simulink model "Project"  (R2018a)
settings: Solver=VariableStepAuto  StartTime=0  StopTime=1  FixedStep=Ts  RelTol=1e-3  AbsTol=1e-3
PreLoadFcn:
  | Ts=2e-6;
  | Ts_Control=100e-6;
undefined symbols (not defined in the file): Hydride, Metal, Nickel, Vnom_dc
libraries: powerlib x111, powerlib_extras x45, simulink x32, powerlib_meascontrol x13, dspswit3 x9, electricdrivelib x2, re_lib x2
(part 1 of 4)
Description:
  | Copyright 2008-2011 The MathWorks, Inc.
settings Model: FPTRunName=Active  ExtModeTrigMode=oneshot  ExtModeArmWhenConnect=off  ExtModeAutoUpdateStatusClock=off  Creator=MathWorks  LastModifiedBy=Lenovo
settings SolverCC: AutoScaleAbsTol=off
settings DataIOCC: SaveFormat=Array  SignalLoggingSaveFormat=ModelDataLogs  SaveOutput=off  SaveTime=off  SignalLoggingName=sigsOut
settings OptimizationCC: BlockReduction=off  BooleanDataType=off  ExpressionDepthLimit=2147483647  InitFltsAndDblsToZero=on  EfficientMapNaN2IntZero=off  LifeSpan=inf
settings DebuggingCC: SaveWithParameterizedLinksMsg=none  UnderspecifiedInitializationDetection=Classic  MergeDetectMultiDrivingBlocksExec=none  CheckExecutionContextPreStartOutputMsg=on  CheckExecutionContextRuntimeOutputMsg=on  SignalResolutionControl=TryResolveAllWithWarning  MultiTaskDSMMsg=warning  MultiTaskCondExecSysMsg=none  FcnCallInpInsideContextMsg=warning  StateNameClashWarn=warning  SFUnexpectedBacktrackingDiag=warning  SFNoUnconditionalDefaultTransitionDiag=warning  SFExecutionAtInitializationDiag=none
settings HardwareCC: ProdBitPerPointer=32  ProdBitPerSizeT=32  ProdBitPerPtrDiffT=32  ProdLargestAtomicFloat=None  ProdIntDivRoundTo=Undefined  ProdEndianess=Unspecified  ProdWordSize=32  ProdHWDeviceType=32-bit Generic  TargetUnknown=on
settings ModelReferenceCC: PropagateSignalLabelsOutOfModel=off
settings CodeAppCC: StateflowObjectComments=on
settings GRTTargetCC: TargetFcnLib=ansi_tfl_tmw.mat  TargetLangStandard=C89/C90 (ANSI)  GeneratePreprocessorConditionals=Disable all  CombineOutputUpdateFcns=off  GRTInterface=on
settings ConfigComp: CovMetricSettings=dw  CovHtmlReporting=on  CovSaveCumulativeToWorkspaceVar=on  CovSaveSingleToWorkspaceVar=on  CovExternalEMLEnable=off
settings SimscapeCC: SimscapeNormalizeSystem=off

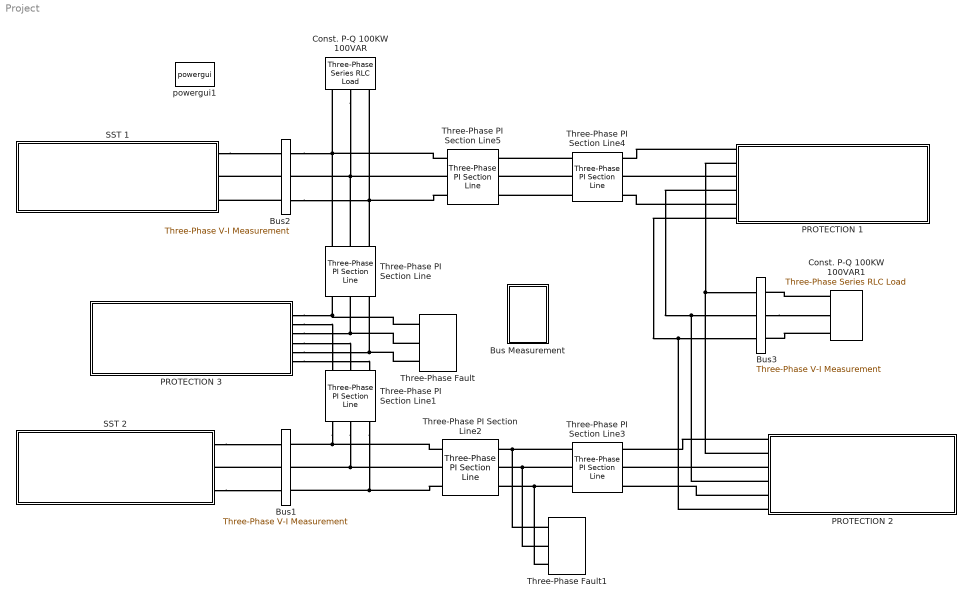
== system Project ==
  Bus Measurement : Subsystem
  Bus1 : powerlib/Measurements/Three-Phase V-I Measurement  VoltageMeasurement=phase-to-phase  SetLabelV=on  LabelV=Bus1_V  Vpu=off  VpuLL=off  CurrentMeasurement=yes  SetLabelI=on  LabelI=Bus1_I  Ipu=off  Pbase=100e6  Vbase=500e3  OutputType=Complex  PhasorSimulation=off  PSBequivalent=0
  Bus2 : powerlib/Measurements/Three-Phase V-I Measurement  VoltageMeasurement=phase-to-phase  SetLabelV=on  LabelV=Bus2_V  Vpu=off  VpuLL=off  CurrentMeasurement=yes  SetLabelI=on  LabelI=Bus2_I  Ipu=off  Pbase=100e6  Vbase=500e3  OutputType=Complex  PhasorSimulation=off  PSBequivalent=0
  Bus3 : powerlib/Measurements/Three-Phase V-I Measurement  VoltageMeasurement=phase-to-phase  SetLabelV=on  LabelV=Bus3_V  Vpu=off  VpuLL=off  CurrentMeasurement=yes  SetLabelI=on  LabelI=Bus3_I  Ipu=off  Pbase=100e6  Vbase=500e3  OutputType=Complex  PhasorSimulation=off  PSBequivalent=0
  Const. P-Q 100KW 100VAR : powerlib/Elements/Three-Phase Series RLC Load  LConnTagsString=A|B|C  Configuration=Y (grounded)  NominalVoltage=380  Vabc=[1e3 1e3 1e3]  Vabcp=[1e3 1e3 1e3]  NominalFrequency=60  UnbalancedPower=off  ActivePower=100e3  InductivePower=100  CapacitivePower=100  Pabc=[10e3 9e3 11e3]  QLabc=[100 90 110]  QCabc=[100 90 110]  Pabcp=[10e3 9e3 11e3]  QLabcp=[100 90 110]  QCabcp=[100 90 110]  Measurements=None  LoadType=constant PQ
  Const. P-Q 100KW 100VAR1 : powerlib/Elements/Three-Phase Series RLC Load  LConnTagsString=A|B|C  Configuration=Y (grounded)  NominalVoltage=380  Vabc=[1e3 1e3 1e3]  Vabcp=[1e3 1e3 1e3]  NominalFrequency=60  UnbalancedPower=off  ActivePower=100e3  InductivePower=100  CapacitivePower=100  Pabc=[10e3 9e3 11e3]  QLabc=[100 90 110]  QCabc=[100 90 110]  Pabcp=[10e3 9e3 11e3]  QLabcp=[100 90 110]  QCabcp=[100 90 110]  Measurements=None  LoadType=constant PQ
  PROTECTION 1 : Subsystem
  PROTECTION 2 : Subsystem
  PROTECTION 3 : Subsystem
  SST 1 : Subsystem
  SST 2 : Subsystem
  Three-Phase PI Section Line{,1..5} (6 alike) : powerlib/Elements/Three-Phase PI Section Line  LConnTagsString=a|b|c  RConnTagsString=A|B|C  Frequency=60  Resistances=[ 0.01273 0.3864]  Inductances="[ 0.9337e-3  4.1264e-3]"  Capacitances=[12.74e-9 7.751e-9]  Length=1
      settings: SourceProductName=Simscape Power Systems
  Three-Phase Fault : powerlib/Elements/Three-Phase Fault  InitialStates=0  FaultA=on  FaultB=on  FaultC=on  GroundFault=on  SwitchTimes=[0.5]  External=off  SwitchStatus=NaN  FaultResistance=0.001  GroundResistance=0.01  SnubberResistance=1e6  SnubberCapacitance=inf  Measurements=None
  Three-Phase Fault1 : powerlib/Elements/Three-Phase Fault  InitialStates=0  FaultA=on  FaultB=on  FaultC=on  GroundFault=on  SwitchTimes=[0.8 0.9]  External=off  SwitchStatus=NaN  FaultResistance=0.001  GroundResistance=0.01  SnubberResistance=1e6  SnubberCapacitance=inf  Measurements=None
  powergui1 : powerlib/powergui  Priority=2  SimulationMode=Discrete  SampleTime=5e-6  frequency=60  Iterations=50  frequencyindice=0  Pbase=100e6  ErrMax=1e-4  UnitsV=kV  UnitsW=MW  buscounter=0  FunctionMessages=off  echomessages=on  EnableUseOfTLC=off  CurrentSourceSwitches=off  DisableSnubberDevices=off  DisableRonSwitches=off  DisableVfSwitches=off  DisplayEquations=off  SolverType=Tustin/Backward Euler (TBE)  Interpol=off  ExternalGateDelay=off  methode=off  Ts=100  x0status=blocks  SPID=off  SwTol=0  HookPort=off  RestoreLinks=warning  ResistiveCurrentMeasurement=off  Frange=[0:2:500]  Ylog=off  Xlog=on  ShowGrid=off  save=off  variable=ZData  structure=psbbridges_str  ZoomFFT=on  StartTime=0.1-2/50  cycles=2  DisplayStyle=off  fundamental=50  FreqAxis=off  MaxFrequency=7000  frequencyindicesteady=1  RmsSteady=1  display=off
  connections:
  Bus2/RConn1 -- Three-Phase PI Section Line/LConn1 -- Three-Phase PI Section Line5/RConn1 -- Const. P-Q 100KW 100VAR/LConn1
  Const. P-Q 100KW 100VAR/LConn2 -- Three-Phase PI Section Line/LConn2 -- Three-Phase PI Section Line5/RConn2 -- Bus2/RConn2
  Bus2/RConn3 -- Three-Phase PI Section Line/LConn3 -- Three-Phase PI Section Line5/RConn3 -- Const. P-Q 100KW 100VAR/LConn3
  SST 1/LConn1 -- Bus2/LConn1
  Bus2/LConn2 -- SST 1/LConn2
  Bus2/LConn3 -- SST 1/LConn3
  SST 2/LConn1 -- Bus1/LConn1
  Bus1/LConn2 -- SST 2/LConn2
  SST 2/LConn3 -- Bus1/LConn3
  Three-Phase PI Section Line1/RConn1 -- Three-Phase PI Section Line2/RConn1 -- Bus1/RConn1
  Three-Phase PI Section Line1/RConn2 -- Three-Phase PI Section Line2/RConn2 -- Bus1/RConn2
  Three-Phase PI Section Line1/RConn3 -- Three-Phase PI Section Line2/RConn3 -- Bus1/RConn3
  Const. P-Q 100KW 100VAR1/LConn1 -- Bus3/RConn1
  Bus3/RConn2 -- Const. P-Q 100KW 100VAR1/LConn2
  Const. P-Q 100KW 100VAR1/LConn3 -- Bus3/RConn3
  Three-Phase PI Section Line4/RConn1 -- Three-Phase PI Section Line5/LConn1
  Three-Phase PI Section Line4/RConn2 -- Three-Phase PI Section Line5/LConn2
  Three-Phase PI Section Line4/RConn3 -- Three-Phase PI Section Line5/LConn3
  Three-Phase PI Section Line3/RConn1 -- Three-Phase Fault1/LConn1 -- Three-Phase PI Section Line2/LConn1
  Three-Phase PI Section Line3/RConn2 -- Three-Phase Fault1/LConn2 -- Three-Phase PI Section Line2/LConn2
  Three-Phase PI Section Line3/RConn3 -- Three-Phase PI Section Line2/LConn3 -- Three-Phase Fault1/LConn3
  PROTECTION 1/LConn1 -- Three-Phase PI Section Line4/LConn1
  PROTECTION 1/LConn3 -- Three-Phase PI Section Line4/LConn2
  PROTECTION 1/LConn5 -- Three-Phase PI Section Line4/LConn3
  PROTECTION 1/LConn2 -- PROTECTION 2/LConn2 -- Bus3/LConn1
  PROTECTION 1/LConn4 -- PROTECTION 2/LConn4 -- Bus3/LConn2
  PROTECTION 1/LConn6 -- PROTECTION 2/LConn6 -- Bus3/LConn3
  PROTECTION 3/LConn1 -- Three-Phase Fault/LConn1 -- Three-Phase PI Section Line/RConn1
  PROTECTION 3/LConn3 -- Three-Phase Fault/LConn2 -- Three-Phase PI Section Line/RConn2
  PROTECTION 3/LConn5 -- Three-Phase Fault/LConn3 -- Three-Phase PI Section Line/RConn3
  PROTECTION 3/LConn2 -- Three-Phase PI Section Line1/LConn1
  PROTECTION 3/LConn4 -- Three-Phase PI Section Line1/LConn2
  PROTECTION 3/LConn6 -- Three-Phase PI Section Line1/LConn3
  PROTECTION 2/LConn1 -- Three-Phase PI Section Line3/LConn1
  PROTECTION 2/LConn3 -- Three-Phase PI Section Line3/LConn2
  PROTECTION 2/LConn5 -- Three-Phase PI Section Line3/LConn3

== system Project/Bus Measurement ==
  Scope{,1..5} (6 alike) : Scope
  wires:
  [Bus3_V] -> Scope4/1
  [Bus2_I] -> Scope3/1
  [Bus2_V] -> Scope2/1
  [Bus1_I] -> Scope1/1
  [Bus3_I] -> Scope5/1
  [Bus1_V] -> Scope/1

== system Project/PROTECTION 1 ==
  Current Measurement : powerlib/Measurements/Current Measurement  PhasorSimulation=off  OutputType=Complex  PSBequivalent=0
  Current Measurement1 : powerlib/Measurements/Current Measurement  PhasorSimulation=off  OutputType=Complex  PSBequivalent=0
  Current Measurement2 : powerlib/Measurements/Current Measurement  PhasorSimulation=off  OutputType=Complex  PSBequivalent=0
  overcurrent Fid : Subsystem
  overcurrent Fid1 : Subsystem
  overcurrent Fid2 : Subsystem
  overcurrent relay1 : Subsystem
  overcurrent relay2 : Subsystem
  overcurrent relay3 : Subsystem
  Conn1 : PMIOPort  Side=Left
  Conn2 : PMIOPort  Port=2  Side=Left
  Conn3 : PMIOPort  Port=3  Side=Left
  Conn4 : PMIOPort  Port=4  Side=Left
  Conn5 : PMIOPort  Port=5  Side=Left
  Conn6 : PMIOPort  Port=6  Side=Left
  wires:
  overcurrent relay1/1("CB control signal ") -> overcurrent Fid/1(In_Rly)
  overcurrent relay2/1("CB control signal ") -> overcurrent Fid2/1(In_Rly)
  overcurrent relay3/1("CB control signal ") -> overcurrent Fid1/1(In_Rly)
  Current Measurement/1 -> overcurrent relay1/1(Current)
  Current Measurement1/1 -> overcurrent relay2/1(Current)
  Current Measurement2/1 -> overcurrent relay3/1(Current)
  connections:
  Current Measurement2/LConn1 -- Conn5/RConn1
  overcurrent Fid1/LConn2 -- Conn6/RConn1
  overcurrent Fid/LConn2 -- Conn2/RConn1
  Current Measurement1/LConn1 -- Conn3/RConn1
  Current Measurement/LConn1 -- Conn1/RConn1
  Current Measurement/RConn1 -- overcurrent Fid/LConn1
  Current Measurement1/RConn1 -- overcurrent Fid2/LConn1
  Conn4/RConn1 -- overcurrent Fid2/LConn2
  Current Measurement2/RConn1 -- overcurrent Fid1/LConn1

== system Project/PROTECTION 2 ==
  Current Measurement : powerlib/Measurements/Current Measurement  PhasorSimulation=off  OutputType=Complex  PSBequivalent=0
  Current Measurement1 : powerlib/Measurements/Current Measurement  PhasorSimulation=off  OutputType=Complex  PSBequivalent=0
  Current Measurement2 : powerlib/Measurements/Current Measurement  PhasorSimulation=off  OutputType=Complex  PSBequivalent=0
  overcurrent Fid : Subsystem
  overcurrent Fid1 : Subsystem
  overcurrent Fid2 : Subsystem
  overcurrent relay1 : Subsystem
  overcurrent relay2 : Subsystem
  overcurrent relay3 : Subsystem
  Conn1 : PMIOPort  Side=Left
  Conn2 : PMIOPort  Port=2  Side=Left
  Conn3 : PMIOPort  Port=3  Side=Left
  Conn4 : PMIOPort  Port=4  Side=Left
  Conn5 : PMIOPort  Port=5  Side=Left
  Conn6 : PMIOPort  Port=6  Side=Left
  wires:
  Current Measurement1/1 -> overcurrent relay2/1(Current)
  overcurrent relay2/1("CB control signal ") -> overcurrent Fid2/1(In_Rly)
  Current Measurement2/1 -> overcurrent relay3/1(Current)
  overcurrent relay3/1("CB control signal ") -> overcurrent Fid1/1(In_Rly)
  Current Measurement/1 -> overcurrent relay1/1(Current)
  overcurrent relay1/1("CB control signal ") -> overcurrent Fid/1(In_Rly)
  connections:
  Current Measurement2/RConn1 -- overcurrent Fid1/LConn1
  overcurrent Fid1/LConn2 -- Conn6/RConn1
  Current Measurement/RConn1 -- overcurrent Fid/LConn1
  Current Measurement2/LConn1 -- Conn5/RConn1
  Current Measurement1/LConn1 -- Conn3/RConn1
  Conn4/RConn1 -- overcurrent Fid2/LConn2
  Current Measurement/LConn1 -- Conn1/RConn1
  Current Measurement1/RConn1 -- overcurrent Fid2/LConn1
  overcurrent Fid/LConn2 -- Conn2/RConn1

== system Project/PROTECTION 3 ==
  Current Measurement : powerlib/Measurements/Current Measurement  PhasorSimulation=off  OutputType=Complex  PSBequivalent=0
  Current Measurement1 : powerlib/Measurements/Current Measurement  PhasorSimulation=off  OutputType=Complex  PSBequivalent=0
  Current Measurement2 : powerlib/Measurements/Current Measurement  PhasorSimulation=off  OutputType=Complex  PSBequivalent=0
  Scope : Scope
  overcurrent Fid : Subsystem
  overcurrent Fid1 : Subsystem
  overcurrent Fid2 : Subsystem
  overcurrent relay1 : Subsystem
  overcurrent relay2 : Subsystem
  overcurrent relay3 : Subsystem
  Conn1 : PMIOPort  Side=Left
  Conn2 : PMIOPort  Port=2  Side=Left
  Conn3 : PMIOPort  Port=3  Side=Left
  Conn4 : PMIOPort  Port=4  Side=Left
  Conn5 : PMIOPort  Port=5  Side=Left
  Conn6 : PMIOPort  Port=6  Side=Left
  wires:
  Current Measurement1/1 -> overcurrent relay2/1(Current)
  overcurrent relay2/1("CB control signal ") -> overcurrent Fid2/1(In_Rly)
  Current Measurement2/1 -> overcurrent relay3/1(Current)
  overcurrent relay3/1("CB control signal ") -> overcurrent Fid1/1(In_Rly)
  Current Measurement/1 -> Scope/1, overcurrent relay1/1(Current)
  overcurrent relay1/1("CB control signal ") -> overcurrent Fid/1(In_Rly)
  connections:
  Current Measurement2/RConn1 -- overcurrent Fid1/LConn1
  overcurrent Fid1/LConn2 -- Conn6/RConn1
  Current Measurement/RConn1 -- overcurrent Fid/LConn1
  Current Measurement2/LConn1 -- Conn5/RConn1
  Current Measurement1/LConn1 -- Conn3/RConn1
  Conn4/RConn1 -- overcurrent Fid2/LConn2
  Current Measurement/LConn1 -- Conn1/RConn1
  Current Measurement1/RConn1 -- overcurrent Fid2/LConn1
  overcurrent Fid/LConn2 -- Conn2/RConn1

== system Project/SST 1 ==
  note: 1=SST
  note: 0=PV
  "6.2 kV, 60 Hz " : powerlib/Electrical Sources/Three-Phase Source  InternalConnection=Yg  VoltagePhases=off  Voltage=6.2e3  PhaseAngle=0  Voltage_phases=[25e3 25e3 25e3]/sqrt(3)  PhaseAngles_phases=[0 -120 +120]  Frequency=60  NonIdealSource=on  SpecifyImpedance=off  Resistance=25e3^2/10e6/5  Inductance=0  ShortCircuitLevel=1e6  BaseVoltage=6.2e3  XRratio=5  BusType=swing  Pref=0  Qref=0  Prefabc=[10e3, 10e3, 10e3]  Qrefabc=[0, 0, 0]  Qmin=-inf  Qmax=inf
  AC-DC Conversion : Subsystem
  Battery (DESD) : Subsystem
  C1 : powerlib/Elements/Parallel RLC Branch  LConnTagsString=a  RConnTagsString=__new0  BranchType=C  Resistance=inf  Inductance=inf  SetiL0=off  InitialCurrent=0  Capacitance=1800e-06  Setx0=off  InitialVoltage=0  Measurements=None
  C2 : powerlib/Elements/Parallel RLC Branch  LConnTagsString=a  RConnTagsString=__new0  BranchType=C  Resistance=inf  Inductance=inf  SetiL0=off  InitialCurrent=0  Capacitance=80e-3  Setx0=off  InitialVoltage=0  Measurements=None
  Constant : Constant
  DC-AC Conversion : Subsystem
  DC-DC Isolation : Subsystem
  PV (DRER) : Subsystem
  Switch : Subsystem
  a : PMIOPort  Side=Left
  b : PMIOPort  Port=2  Side=Left
  c : PMIOPort  Port=3  Side=Left
  wires:
  Constant/1 -> Switch/1(In1)
  connections:
  AC-DC Conversion/RConn1 -- C1/LConn1 -- DC-DC Isolation/RConn1
  "6.2 kV, 60 Hz "/RConn2 -- AC-DC Conversion/LConn2
  c/RConn1 -- DC-AC Conversion/LConn3
  DC-AC Conversion/RConn2 -- PV (DRER)/LConn2 -- DC-DC Isolation/LConn2 -- Battery (DESD)/LConn1 -- C2/RConn1
  "6.2 kV, 60 Hz "/RConn3 -- AC-DC Conversion/LConn3
  Switch/LConn1 -- PV (DRER)/LConn1
  C2/LConn1 -- Switch/RConn1 -- Battery (DESD)/RConn1 -- DC-AC Conversion/RConn1
  "6.2 kV, 60 Hz "/RConn1 -- AC-DC Conversion/LConn1
  DC-DC Isolation/RConn2 -- C1/RConn1 -- AC-DC Conversion/RConn2
  Switch/LConn2 -- DC-DC Isolation/LConn1
  DC-AC Conversion/LConn1 -- a/RConn1
  b/RConn1 -- DC-AC Conversion/LConn2

== system Project/SST 2 ==
  note: 1=SST
  note: 0=PV
  "6.2 kV, 60 Hz 1" : powerlib/Electrical Sources/Three-Phase Source  InternalConnection=Yg  VoltagePhases=off  Voltage=6.2e3  PhaseAngle=0  Voltage_phases=[25e3 25e3 25e3]/sqrt(3)  PhaseAngles_phases=[0 -120 +120]  Frequency=60  NonIdealSource=on  SpecifyImpedance=off  Resistance=25e3^2/10e6/5  Inductance=0  ShortCircuitLevel=1e6  BaseVoltage=6.2e3  XRratio=5  BusType=swing  Pref=0  Qref=0  Prefabc=[10e3, 10e3, 10e3]  Qrefabc=[0, 0, 0]  Qmin=-inf  Qmax=inf
  AC-DC Conversion1 : Subsystem
  Battery (DESD)1 : Subsystem
  C3 : powerlib/Elements/Parallel RLC Branch  LConnTagsString=a  RConnTagsString=__new0  BranchType=C  Resistance=inf  Inductance=inf  SetiL0=off  InitialCurrent=0  Capacitance=1800e-06  Setx0=off  InitialVoltage=0  Measurements=None
  C4 : powerlib/Elements/Parallel RLC Branch  LConnTagsString=a  RConnTagsString=__new0  BranchType=C  Resistance=inf  Inductance=inf  SetiL0=off  InitialCurrent=0  Capacitance=80e-3  Setx0=off  InitialVoltage=0  Measurements=None
  Constant1 : Constant
  DC-AC Conversion1 : Subsystem
  DC-DC Isolation1 : Subsystem
  PV (DRER)1 : Subsystem
  Switch1 : Subsystem
  a : PMIOPort  Side=Left
  b : PMIOPort  Port=2  Side=Left
  c : PMIOPort  Port=3  Side=Left
  wires:
  Constant1/1 -> Switch1/1(In1)
  connections:
  C4/RConn1 -- DC-AC Conversion1/RConn2 -- PV (DRER)1/LConn2 -- DC-DC Isolation1/LConn2 -- Battery (DESD)1/LConn1
  AC-DC Conversion1/LConn3 -- "6.2 kV, 60 Hz 1"/RConn3
  "6.2 kV, 60 Hz 1"/RConn2 -- AC-DC Conversion1/LConn2
  Switch1/LConn2 -- DC-DC Isolation1/LConn1
  AC-DC Conversion1/RConn2 -- DC-DC Isolation1/RConn2 -- C3/RConn1
  Switch1/LConn1 -- PV (DRER)1/LConn1
  "6.2 kV, 60 Hz 1"/RConn1 -- AC-DC Conversion1/LConn1
  DC-AC Conversion1/RConn1 -- C4/LConn1 -- Switch1/RConn1 -- Battery (DESD)1/RConn1
  DC-DC Isolation1/RConn1 -- AC-DC Conversion1/RConn1 -- C3/LConn1
  DC-AC Conversion1/LConn1 -- a/RConn1
  DC-AC Conversion1/LConn3 -- c/RConn1
  b/RConn1 -- DC-AC Conversion1/LConn2

== system Project/PROTECTION 1/overcurrent Fid ==
  In_Rly : Inport
  Diode1 : powerlib/Power Electronics/Diode  Ron=0.001  Lon=0  Vf=1  IC=150  UseSnubber=0  Rs=500  Cs=250e-9  Measurements=off
  Diode2 : powerlib/Power Electronics/Diode  Ron=0.001  Lon=0  Vf=1  IC=150  UseSnubber=0  Rs=500  Cs=250e-9  Measurements=off
  IGBT1 : powerlib/Power Electronics/IGBT  Ron=0.001  Lon=100e-6  Vf=3  Tf=1e-6  Tt=2e-6  IC=150  Rs=1e5  Cs=inf  Measurements=on
  IGBT2 : powerlib/Power Electronics/IGBT  Ron=0.001  Lon=100e-6  Vf=3  Tf=1e-6  Tt=2e-6  IC=150  Rs=1e5  Cs=inf  Measurements=on
  Scope : Scope  NumInputPorts=2
  In : PMIOPort  Tag=PMCPort  Side=Left
  Out : PMIOPort  Tag=PMCPort  Port=2  Side=Left
  wires:
  IGBT1/1 -> [igbt1]
  [igbt1] -> Scope/2
  In_Rly/1 -> IGBT1/1, IGBT2/1
  IGBT2/1 -> [igbt]
  [igbt] -> Scope/1
  connections:
  IGBT2/RConn1 -- Diode2/LConn1 -- IGBT1/RConn1 -- Diode1/LConn1
  In/RConn1 -- Diode1/RConn1 -- IGBT2/LConn1
  Out/RConn1 -- Diode2/RConn1 -- IGBT1/LConn1

== system Project/PROTECTION 1/overcurrent Fid1 ==
  In_Rly : Inport
  Diode1 : powerlib/Power Electronics/Diode  Ron=0.001  Lon=0  Vf=1  IC=150  UseSnubber=0  Rs=500  Cs=250e-9  Measurements=off
  Diode2 : powerlib/Power Electronics/Diode  Ron=0.001  Lon=0  Vf=1  IC=150  UseSnubber=0  Rs=500  Cs=250e-9  Measurements=off
  IGBT1 : powerlib/Power Electronics/IGBT  Ron=0.001  Lon=100e-6  Vf=3  Tf=1e-6  Tt=2e-6  IC=150  Rs=1e5  Cs=inf  Measurements=on
  IGBT2 : powerlib/Power Electronics/IGBT  Ron=0.001  Lon=100e-6  Vf=3  Tf=1e-6  Tt=2e-6  IC=150  Rs=1e5  Cs=inf  Measurements=on
  Scope : Scope  NumInputPorts=2
  In : PMIOPort  Tag=PMCPort  Side=Left
  Out : PMIOPort  Tag=PMCPort  Port=2  Side=Left
  wires:
  [igbt] -> Scope/1
  IGBT2/1 -> [igbt]
  In_Rly/1 -> IGBT2/1, IGBT1/1
  [igbt1] -> Scope/2
  IGBT1/1 -> [igbt1]
  connections:
  IGBT1/LConn1 -- Diode2/RConn1 -- Out/RConn1
  IGBT2/LConn1 -- Diode1/RConn1 -- In/RConn1
  Diode1/LConn1 -- IGBT1/RConn1 -- Diode2/LConn1 -- IGBT2/RConn1

== system Project/PROTECTION 1/overcurrent Fid2 ==
  In_Rly : Inport
  Diode1 : powerlib/Power Electronics/Diode  Ron=0.001  Lon=0  Vf=1  IC=150  UseSnubber=0  Rs=500  Cs=250e-9  Measurements=off
  Diode2 : powerlib/Power Electronics/Diode  Ron=0.001  Lon=0  Vf=1  IC=150  UseSnubber=0  Rs=500  Cs=250e-9  Measurements=off
  IGBT1 : powerlib/Power Electronics/IGBT  Ron=0.001  Lon=100e-6  Vf=3  Tf=1e-6  Tt=2e-6  IC=150  Rs=1e5  Cs=inf  Measurements=on
  IGBT2 : powerlib/Power Electronics/IGBT  Ron=0.001  Lon=100e-6  Vf=3  Tf=1e-6  Tt=2e-6  IC=150  Rs=1e5  Cs=inf  Measurements=on
  Scope : Scope  NumInputPorts=2
  In : PMIOPort  Tag=PMCPort  Side=Left
  Out : PMIOPort  Tag=PMCPort  Port=2  Side=Left
  wires:
  [igbt] -> Scope/1
  IGBT2/1 -> [igbt]
  In_Rly/1 -> IGBT2/1, IGBT1/1
  [igbt1] -> Scope/2
  IGBT1/1 -> [igbt1]
  connections:
  IGBT1/LConn1 -- Diode2/RConn1 -- Out/RConn1
  IGBT2/LConn1 -- Diode1/RConn1 -- In/RConn1
  Diode1/LConn1 -- IGBT1/RConn1 -- Diode2/LConn1 -- IGBT2/RConn1

== system Project/PROTECTION 1/overcurrent relay1 ==
  Current : Inport
  Constant : Constant
  Constant2 : Constant  Value=0
  Counter1 : dspswit3/Counter  Direction=Up  CountEvent=Rising edge  CounterSize=8 bits  MaxCount=255  InitialCount=0  Output=Count and Hit  HitValue=1  ResetInput=off  SamplesPerFrame=1  Ts=1  CntDtype=double  HitDtype=Logical
  Data  Conversion : DataTypeConversion  OutDataTypeStr=double
  Delay : Delay  DelayLength=1
  Display{2..6} (5 alike) : Display
  Main Relay : Subsystem
  Monostable : powerlib_meascontrol/Logic/Monostable  EdgeDetect=Rising  PulseDuration=.05  ic=0  Ts=0
      settings: SourceProductName=Simscape Power Systems  SourceProductBaseCode=PS
  Not{1,3..5} (4 alike) : Logic  Operator=NOT  IconShape=distinctive  AllPortsSameDT=off  OutDataTypeStr=boolean
  Scope2 : Scope
  Scope3 : Scope
  Sum : Sum  Inputs=|++
  Switch : Switch  Criteria=u2 > Threshold  Threshold=1
  Switch1 : Switch  Criteria=u2 > Threshold
  "CB control signal " : Outport
  wires:
  Switch/1 -> Display4/1, Not4/1
  Delay/1 -> Sum/2
  Monostable/1 -> Not5/1
  Main Relay/1(AR signal) -> Data  Conversion/1
  Counter1/2 -> Not3/1, Display2/1
  Current/1 -> Main Relay/1("Three phase actual currents ")
  Constant2/1 -> Switch1/3
  Not4/1 -> Monostable/1
  Not3/1 -> Switch1/2, Switch/1
  Counter1/1 -> Switch/2, Display3/1
  Data  Conversion/1 -> Sum/1, Display5/1, Switch/3, Display6/1, Scope3/1
  Not1/1 -> Delay/1
  Not5/1 -> Switch1/1
  Sum/1 -> Counter1/1
  Switch1/1 -> "CB control signal "/1, Scope2/1, Not1/1
  Constant/1 -> Main Relay/2("CT ratio ")

== system Project/PROTECTION 1/overcurrent relay2 ==
  Current : Inport
  Constant : Constant
  Constant2 : Constant  Value=0
  Counter1 : dspswit3/Counter  Direction=Up  CountEvent=Rising edge  CounterSize=8 bits  MaxCount=255  InitialCount=0  Output=Count and Hit  HitValue=1  ResetInput=off  SamplesPerFrame=1  Ts=1  CntDtype=double  HitDtype=Logical
  Data  Conversion : DataTypeConversion  OutDataTypeStr=double
  Delay : Delay  DelayLength=1
  Display{2..6} (5 alike) : Display
  Main Relay : Subsystem
  Monostable : powerlib_meascontrol/Logic/Monostable  EdgeDetect=Rising  PulseDuration=.05  ic=0  Ts=0
      settings: SourceProductName=Simscape Power Systems  SourceProductBaseCode=PS
  Not{1,3..5} (4 alike) : Logic  Operator=NOT  IconShape=distinctive  AllPortsSameDT=off  OutDataTypeStr=boolean
  Scope2 : Scope
  Scope3 : Scope
  Sum : Sum  Inputs=|++
  Switch : Switch  Criteria=u2 > Threshold  Threshold=1
  Switch1 : Switch  Criteria=u2 > Threshold
  "CB control signal " : Outport
  wires:
  Constant/1 -> Main Relay/2("CT ratio ")
  Switch1/1 -> Not1/1, Scope2/1, "CB control signal "/1
  Sum/1 -> Counter1/1
  Not5/1 -> Switch1/1
  Not1/1 -> Delay/1
  Data  Conversion/1 -> Scope3/1, Display6/1, Switch/3, Display5/1, Sum/1
  Counter1/1 -> Display3/1, Switch/2
  Not3/1 -> Switch/1, Switch1/2
  Not4/1 -> Monostable/1
  Constant2/1 -> Switch1/3
  Current/1 -> Main Relay/1("Three phase actual currents ")
  Counter1/2 -> Display2/1, Not3/1
  Main Relay/1(AR signal) -> Data  Conversion/1
  Monostable/1 -> Not5/1
  Delay/1 -> Sum/2
  Switch/1 -> Not4/1, Display4/1

== system Project/PROTECTION 1/overcurrent relay3 ==
  Current : Inport
  Constant : Constant
  Constant2 : Constant  Value=0
  Counter1 : dspswit3/Counter  Direction=Up  CountEvent=Rising edge  CounterSize=8 bits  MaxCount=255  InitialCount=0  Output=Count and Hit  HitValue=1  ResetInput=off  SamplesPerFrame=1  Ts=1  CntDtype=double  HitDtype=Logical
  Data  Conversion : DataTypeConversion  OutDataTypeStr=double
  Delay : Delay  DelayLength=1
  Display{2..6} (5 alike) : Display
  Main Relay : Subsystem
  Monostable : powerlib_meascontrol/Logic/Monostable  EdgeDetect=Rising  PulseDuration=.05  ic=0  Ts=0
      settings: SourceProductName=Simscape Power Systems  SourceProductBaseCode=PS
  Not{1,3..5} (4 alike) : Logic  Operator=NOT  IconShape=distinctive  AllPortsSameDT=off  OutDataTypeStr=boolean
  Scope2 : Scope
  Scope3 : Scope
  Sum : Sum  Inputs=|++
  Switch : Switch  Criteria=u2 > Threshold  Threshold=1
  Switch1 : Switch  Criteria=u2 > Threshold
  "CB control signal " : Outport
  wires:
  Constant/1 -> Main Relay/2("CT ratio ")
  Switch1/1 -> Not1/1, Scope2/1, "CB control signal "/1
  Sum/1 -> Counter1/1
  Not5/1 -> Switch1/1
  Not1/1 -> Delay/1
  Data  Conversion/1 -> Scope3/1, Display6/1, Switch/3, Display5/1, Sum/1
  Counter1/1 -> Display3/1, Switch/2
  Not3/1 -> Switch/1, Switch1/2
  Not4/1 -> Monostable/1
  Constant2/1 -> Switch1/3
  Current/1 -> Main Relay/1("Three phase actual currents ")
  Counter1/2 -> Display2/1, Not3/1
  Main Relay/1(AR signal) -> Data  Conversion/1
  Monostable/1 -> Not5/1
  Delay/1 -> Sum/2
  Switch/1 -> Not4/1, Display4/1

== system Project/PROTECTION 2/overcurrent Fid ==
  In_Rly : Inport
  Diode1 : powerlib/Power Electronics/Diode  Ron=0.001  Lon=0  Vf=1  IC=150  UseSnubber=0  Rs=500  Cs=250e-9  Measurements=off
  Diode2 : powerlib/Power Electronics/Diode  Ron=0.001  Lon=0  Vf=1  IC=150  UseSnubber=0  Rs=500  Cs=250e-9  Measurements=off
  IGBT1 : powerlib/Power Electronics/IGBT  Ron=0.001  Lon=100e-6  Vf=3  Tf=1e-6  Tt=2e-6  IC=150  Rs=1e5  Cs=inf  Measurements=on
  IGBT2 : powerlib/Power Electronics/IGBT  Ron=0.001  Lon=100e-6  Vf=3  Tf=1e-6  Tt=2e-6  IC=150  Rs=1e5  Cs=inf  Measurements=on
  Scope : Scope  NumInputPorts=2
  In : PMIOPort  Tag=PMCPort  Side=Left
  Out : PMIOPort  Tag=PMCPort  Port=2  Side=Left
  wires:
  IGBT1/1 -> [igbt1]
  [igbt1] -> Scope/2
  In_Rly/1 -> IGBT1/1, IGBT2/1
  IGBT2/1 -> [igbt]
  [igbt] -> Scope/1
  connections:
  IGBT2/RConn1 -- Diode2/LConn1 -- IGBT1/RConn1 -- Diode1/LConn1
  In/RConn1 -- Diode1/RConn1 -- IGBT2/LConn1
  Out/RConn1 -- Diode2/RConn1 -- IGBT1/LConn1

== system Project/PROTECTION 2/overcurrent Fid1 ==
  In_Rly : Inport
  Diode1 : powerlib/Power Electronics/Diode  Ron=0.001  Lon=0  Vf=1  IC=150  UseSnubber=0  Rs=500  Cs=250e-9  Measurements=off
  Diode2 : powerlib/Power Electronics/Diode  Ron=0.001  Lon=0  Vf=1  IC=150  UseSnubber=0  Rs=500  Cs=250e-9  Measurements=off
  IGBT1 : powerlib/Power Electronics/IGBT  Ron=0.001  Lon=100e-6  Vf=3  Tf=1e-6  Tt=2e-6  IC=150  Rs=1e5  Cs=inf  Measurements=on
  IGBT2 : powerlib/Power Electronics/IGBT  Ron=0.001  Lon=100e-6  Vf=3  Tf=1e-6  Tt=2e-6  IC=150  Rs=1e5  Cs=inf  Measurements=on
  Scope : Scope  NumInputPorts=2
  In : PMIOPort  Tag=PMCPort  Side=Left
  Out : PMIOPort  Tag=PMCPort  Port=2  Side=Left
  wires:
  [igbt] -> Scope/1
  IGBT2/1 -> [igbt]
  In_Rly/1 -> IGBT2/1, IGBT1/1
  [igbt1] -> Scope/2
  IGBT1/1 -> [igbt1]
  connections:
  IGBT1/LConn1 -- Diode2/RConn1 -- Out/RConn1
  IGBT2/LConn1 -- Diode1/RConn1 -- In/RConn1
  Diode1/LConn1 -- IGBT1/RConn1 -- Diode2/LConn1 -- IGBT2/RConn1

== system Project/PROTECTION 2/overcurrent Fid2 ==
  In_Rly : Inport
  Diode1 : powerlib/Power Electronics/Diode  Ron=0.001  Lon=0  Vf=1  IC=150  UseSnubber=0  Rs=500  Cs=250e-9  Measurements=off
  Diode2 : powerlib/Power Electronics/Diode  Ron=0.001  Lon=0  Vf=1  IC=150  UseSnubber=0  Rs=500  Cs=250e-9  Measurements=off
  IGBT1 : powerlib/Power Electronics/IGBT  Ron=0.001  Lon=100e-6  Vf=3  Tf=1e-6  Tt=2e-6  IC=150  Rs=1e5  Cs=inf  Measurements=on
  IGBT2 : powerlib/Power Electronics/IGBT  Ron=0.001  Lon=100e-6  Vf=3  Tf=1e-6  Tt=2e-6  IC=150  Rs=1e5  Cs=inf  Measurements=on
  Scope : Scope  NumInputPorts=2
  In : PMIOPort  Tag=PMCPort  Side=Left
  Out : PMIOPort  Tag=PMCPort  Port=2  Side=Left
  wires:
  [igbt] -> Scope/1
  IGBT2/1 -> [igbt]
  In_Rly/1 -> IGBT2/1, IGBT1/1
  [igbt1] -> Scope/2
  IGBT1/1 -> [igbt1]
  connections:
  IGBT1/LConn1 -- Diode2/RConn1 -- Out/RConn1
  IGBT2/LConn1 -- Diode1/RConn1 -- In/RConn1
  Diode1/LConn1 -- IGBT1/RConn1 -- Diode2/LConn1 -- IGBT2/RConn1

== system Project/PROTECTION 2/overcurrent relay1 ==
  Current : Inport
  Constant : Constant
  Constant2 : Constant  Value=0
  Counter1 : dspswit3/Counter  Direction=Up  CountEvent=Rising edge  CounterSize=8 bits  MaxCount=255  InitialCount=0  Output=Count and Hit  HitValue=1  ResetInput=off  SamplesPerFrame=1  Ts=1  CntDtype=double  HitDtype=Logical
  Data  Conversion : DataTypeConversion  OutDataTypeStr=double
  Delay : Delay  DelayLength=1
  Display{2..6} (5 alike) : Display
  Main Relay : Subsystem
  Monostable : powerlib_meascontrol/Logic/Monostable  EdgeDetect=Rising  PulseDuration=.05  ic=0  Ts=0
      settings: SourceProductName=Simscape Power Systems  SourceProductBaseCode=PS
  Not{1,3..5} (4 alike) : Logic  Operator=NOT  IconShape=distinctive  AllPortsSameDT=off  OutDataTypeStr=boolean
  Scope2 : Scope
  Scope3 : Scope
  Sum : Sum  Inputs=|++
  Switch : Switch  Criteria=u2 > Threshold  Threshold=1
  Switch1 : Switch  Criteria=u2 > Threshold
  "CB control signal " : Outport
  wires:
  Switch/1 -> Display4/1, Not4/1
  Delay/1 -> Sum/2
  Monostable/1 -> Not5/1
  Main Relay/1(AR signal) -> Data  Conversion/1
  Counter1/2 -> Not3/1, Display2/1
  Current/1 -> Main Relay/1("Three phase actual currents ")
  Constant2/1 -> Switch1/3
  Not4/1 -> Monostable/1
  Not3/1 -> Switch1/2, Switch/1
  Counter1/1 -> Switch/2, Display3/1
  Data  Conversion/1 -> Sum/1, Display5/1, Switch/3, Display6/1, Scope3/1
  Not1/1 -> Delay/1
  Not5/1 -> Switch1/1
  Sum/1 -> Counter1/1
  Switch1/1 -> "CB control signal "/1, Scope2/1, Not1/1
  Constant/1 -> Main Relay/2("CT ratio ")

== system Project/PROTECTION 2/overcurrent relay2 ==
  Current : Inport
  Constant : Constant
  Constant2 : Constant  Value=0
  Counter1 : dspswit3/Counter  Direction=Up  CountEvent=Rising edge  CounterSize=8 bits  MaxCount=255  InitialCount=0  Output=Count and Hit  HitValue=1  ResetInput=off  SamplesPerFrame=1  Ts=1  CntDtype=double  HitDtype=Logical
  Data  Conversion : DataTypeConversion  OutDataTypeStr=double
  Delay : Delay  DelayLength=1
  Display{2..6} (5 alike) : Display
  Main Relay : Subsystem
  Monostable : powerlib_meascontrol/Logic/Monostable  EdgeDetect=Rising  PulseDuration=.05  ic=0  Ts=0
      settings: SourceProductName=Simscape Power Systems  SourceProductBaseCode=PS
  Not{1,3..5} (4 alike) : Logic  Operator=NOT  IconShape=distinctive  AllPortsSameDT=off  OutDataTypeStr=boolean
  Scope2 : Scope
  Scope3 : Scope
  Sum : Sum  Inputs=|++
  Switch : Switch  Criteria=u2 > Threshold  Threshold=1
  Switch1 : Switch  Criteria=u2 > Threshold
  "CB control signal " : Outport
  wires:
  Constant/1 -> Main Relay/2("CT ratio ")
  Switch1/1 -> Not1/1, Scope2/1, "CB control signal "/1
  Sum/1 -> Counter1/1
  Not5/1 -> Switch1/1
  Not1/1 -> Delay/1
  Data  Conversion/1 -> Scope3/1, Display6/1, Switch/3, Display5/1, Sum/1
  Counter1/1 -> Display3/1, Switch/2
  Not3/1 -> Switch/1, Switch1/2
  Not4/1 -> Monostable/1
  Constant2/1 -> Switch1/3
  Current/1 -> Main Relay/1("Three phase actual currents ")
  Counter1/2 -> Display2/1, Not3/1
  Main Relay/1(AR signal) -> Data  Conversion/1
  Monostable/1 -> Not5/1
  Delay/1 -> Sum/2
  Switch/1 -> Not4/1, Display4/1

== system Project/PROTECTION 2/overcurrent relay3 ==
  Current : Inport
  Constant : Constant
  Constant2 : Constant  Value=0
  Counter1 : dspswit3/Counter  Direction=Up  CountEvent=Rising edge  CounterSize=8 bits  MaxCount=255  InitialCount=0  Output=Count and Hit  HitValue=1  ResetInput=off  SamplesPerFrame=1  Ts=1  CntDtype=double  HitDtype=Logical
  Data  Conversion : DataTypeConversion  OutDataTypeStr=double
  Delay : Delay  DelayLength=1
  Display{2..6} (5 alike) : Display
  Main Relay : Subsystem
  Monostable : powerlib_meascontrol/Logic/Monostable  EdgeDetect=Rising  PulseDuration=.05  ic=0  Ts=0
      settings: SourceProductName=Simscape Power Systems  SourceProductBaseCode=PS
  Not{1,3..5} (4 alike) : Logic  Operator=NOT  IconShape=distinctive  AllPortsSameDT=off  OutDataTypeStr=boolean
  Scope2 : Scope
  Scope3 : Scope
  Sum : Sum  Inputs=|++
  Switch : Switch  Criteria=u2 > Threshold  Threshold=1
  Switch1 : Switch  Criteria=u2 > Threshold
  "CB control signal " : Outport
  wires:
  Constant/1 -> Main Relay/2("CT ratio ")
  Switch1/1 -> Not1/1, Scope2/1, "CB control signal "/1
  Sum/1 -> Counter1/1
  Not5/1 -> Switch1/1
  Not1/1 -> Delay/1
  Data  Conversion/1 -> Scope3/1, Display6/1, Switch/3, Display5/1, Sum/1
  Counter1/1 -> Display3/1, Switch/2
  Not3/1 -> Switch/1, Switch1/2
  Not4/1 -> Monostable/1
  Constant2/1 -> Switch1/3
  Current/1 -> Main Relay/1("Three phase actual currents ")
  Counter1/2 -> Display2/1, Not3/1
  Main Relay/1(AR signal) -> Data  Conversion/1
  Monostable/1 -> Not5/1
  Delay/1 -> Sum/2
  Switch/1 -> Not4/1, Display4/1

== system Project/PROTECTION 3/overcurrent Fid ==
  In_Rly : Inport
  Diode1 : powerlib/Power Electronics/Diode  Ron=0.001  Lon=0  Vf=1  IC=150  UseSnubber=0  Rs=500  Cs=250e-9  Measurements=off
  Diode2 : powerlib/Power Electronics/Diode  Ron=0.001  Lon=0  Vf=1  IC=150  UseSnubber=0  Rs=500  Cs=250e-9  Measurements=off
  IGBT1 : powerlib/Power Electronics/IGBT  Ron=0.001  Lon=100e-6  Vf=3  Tf=1e-6  Tt=2e-6  IC=150  Rs=1e5  Cs=inf  Measurements=on
  IGBT2 : powerlib/Power Electronics/IGBT  Ron=0.001  Lon=100e-6  Vf=3  Tf=1e-6  Tt=2e-6  IC=150  Rs=1e5  Cs=inf  Measurements=on
  Scope : Scope  NumInputPorts=2
  In : PMIOPort  Tag=PMCPort  Side=Left
  Out : PMIOPort  Tag=PMCPort  Port=2  Side=Left
  wires:
  IGBT1/1 -> [igbt1]
  [igbt1] -> Scope/2
  In_Rly/1 -> IGBT1/1, IGBT2/1
  IGBT2/1 -> [igbt]
  [igbt] -> Scope/1
  connections:
  IGBT2/RConn1 -- Diode2/LConn1 -- IGBT1/RConn1 -- Diode1/LConn1
  In/RConn1 -- Diode1/RConn1 -- IGBT2/LConn1
  Out/RConn1 -- Diode2/RConn1 -- IGBT1/LConn1

== system Project/PROTECTION 3/overcurrent Fid1 ==
  In_Rly : Inport
  Diode1 : powerlib/Power Electronics/Diode  Ron=0.001  Lon=0  Vf=1  IC=150  UseSnubber=0  Rs=500  Cs=250e-9  Measurements=off
  Diode2 : powerlib/Power Electronics/Diode  Ron=0.001  Lon=0  Vf=1  IC=150  UseSnubber=0  Rs=500  Cs=250e-9  Measurements=off
  IGBT1 : powerlib/Power Electronics/IGBT  Ron=0.001  Lon=100e-6  Vf=3  Tf=1e-6  Tt=2e-6  IC=150  Rs=1e5  Cs=inf  Measurements=on
  IGBT2 : powerlib/Power Electronics/IGBT  Ron=0.001  Lon=100e-6  Vf=3  Tf=1e-6  Tt=2e-6  IC=150  Rs=1e5  Cs=inf  Measurements=on
  Scope : Scope  NumInputPorts=2
  In : PMIOPort  Tag=PMCPort  Side=Left
  Out : PMIOPort  Tag=PMCPort  Port=2  Side=Left
  wires:
  [igbt] -> Scope/1
  IGBT2/1 -> [igbt]
  In_Rly/1 -> IGBT2/1, IGBT1/1
  [igbt1] -> Scope/2
  IGBT1/1 -> [igbt1]
  connections:
  IGBT1/LConn1 -- Diode2/RConn1 -- Out/RConn1
  IGBT2/LConn1 -- Diode1/RConn1 -- In/RConn1
  Diode1/LConn1 -- IGBT1/RConn1 -- Diode2/LConn1 -- IGBT2/RConn1

== system Project/PROTECTION 3/overcurrent Fid2 ==
  In_Rly : Inport
  Diode1 : powerlib/Power Electronics/Diode  Ron=0.001  Lon=0  Vf=1  IC=150  UseSnubber=0  Rs=500  Cs=250e-9  Measurements=off
  Diode2 : powerlib/Power Electronics/Diode  Ron=0.001  Lon=0  Vf=1  IC=150  UseSnubber=0  Rs=500  Cs=250e-9  Measurements=off
  IGBT1 : powerlib/Power Electronics/IGBT  Ron=0.001  Lon=100e-6  Vf=3  Tf=1e-6  Tt=2e-6  IC=150  Rs=1e5  Cs=inf  Measurements=on
  IGBT2 : powerlib/Power Electronics/IGBT  Ron=0.001  Lon=100e-6  Vf=3  Tf=1e-6  Tt=2e-6  IC=150  Rs=1e5  Cs=inf  Measurements=on
  Scope : Scope  NumInputPorts=2
  In : PMIOPort  Tag=PMCPort  Side=Left
  Out : PMIOPort  Tag=PMCPort  Port=2  Side=Left
  wires:
  [igbt] -> Scope/1
  IGBT2/1 -> [igbt]
  In_Rly/1 -> IGBT2/1, IGBT1/1
  [igbt1] -> Scope/2
  IGBT1/1 -> [igbt1]
  connections:
  IGBT1/LConn1 -- Diode2/RConn1 -- Out/RConn1
  IGBT2/LConn1 -- Diode1/RConn1 -- In/RConn1
  Diode1/LConn1 -- IGBT1/RConn1 -- Diode2/LConn1 -- IGBT2/RConn1

== system Project/PROTECTION 3/overcurrent relay1 ==
  Current : Inport
  Constant : Constant
  Constant2 : Constant  Value=0
  Counter1 : dspswit3/Counter  Direction=Up  CountEvent=Rising edge  CounterSize=8 bits  MaxCount=255  InitialCount=0  Output=Count and Hit  HitValue=1  ResetInput=off  SamplesPerFrame=1  Ts=1  CntDtype=double  HitDtype=Logical
  Data  Conversion : DataTypeConversion  OutDataTypeStr=double
  Delay : Delay  DelayLength=1
  Display{2..6} (5 alike) : Display
  Main Relay : Subsystem
  Monostable : powerlib_meascontrol/Logic/Monostable  EdgeDetect=Rising  PulseDuration=.05  ic=0  Ts=0
      settings: SourceProductName=Simscape Power Systems  SourceProductBaseCode=PS
  Not{1,3..5} (4 alike) : Logic  Operator=NOT  IconShape=distinctive  AllPortsSameDT=off  OutDataTypeStr=boolean
  Scope2 : Scope
  Scope3 : Scope
  Sum : Sum  Inputs=|++
  Switch : Switch  Criteria=u2 > Threshold  Threshold=1
  Switch1 : Switch  Criteria=u2 > Threshold
  "CB control signal " : Outport
  wires:
  Switch/1 -> Display4/1, Not4/1
  Delay/1 -> Sum/2
  Monostable/1 -> Not5/1
  Main Relay/1(AR signal) -> Data  Conversion/1
  Counter1/2 -> Not3/1, Display2/1
  Current/1 -> Main Relay/1("Three phase actual currents ")
  Constant2/1 -> Switch1/3
  Not4/1 -> Monostable/1
  Not3/1 -> Switch1/2, Switch/1
  Counter1/1 -> Switch/2, Display3/1
  Data  Conversion/1 -> Sum/1, Display5/1, Switch/3, Display6/1, Scope3/1
  Not1/1 -> Delay/1
  Not5/1 -> Switch1/1
  Sum/1 -> Counter1/1
  Switch1/1 -> "CB control signal "/1, Scope2/1, Not1/1
  Constant/1 -> Main Relay/2("CT ratio ")

== system Project/PROTECTION 3/overcurrent relay2 ==
  Current : Inport
  Constant : Constant
  Constant2 : Constant  Value=0
  Counter1 : dspswit3/Counter  Direction=Up  CountEvent=Rising edge  CounterSize=8 bits  MaxCount=255  InitialCount=0  Output=Count and Hit  HitValue=1  ResetInput=off  SamplesPerFrame=1  Ts=1  CntDtype=double  HitDtype=Logical
  Data  Conversion : DataTypeConversion  OutDataTypeStr=double
  Delay : Delay  DelayLength=1
  Display{2..6} (5 alike) : Display
  Main Relay : Subsystem
  Monostable : powerlib_meascontrol/Logic/Monostable  EdgeDetect=Rising  PulseDuration=.05  ic=0  Ts=0
      settings: SourceProductName=Simscape Power Systems  SourceProductBaseCode=PS
  Not{1,3..5} (4 alike) : Logic  Operator=NOT  IconShape=distinctive  AllPortsSameDT=off  OutDataTypeStr=boolean
  Scope2 : Scope
  Scope3 : Scope
  Sum : Sum  Inputs=|++
  Switch : Switch  Criteria=u2 > Threshold  Threshold=1
  Switch1 : Switch  Criteria=u2 > Threshold
  "CB control signal " : Outport
  wires:
  Constant/1 -> Main Relay/2("CT ratio ")
  Switch1/1 -> Not1/1, Scope2/1, "CB control signal "/1
  Sum/1 -> Counter1/1
  Not5/1 -> Switch1/1
  Not1/1 -> Delay/1
  Data  Conversion/1 -> Scope3/1, Display6/1, Switch/3, Display5/1, Sum/1
  Counter1/1 -> Display3/1, Switch/2
  Not3/1 -> Switch/1, Switch1/2
  Not4/1 -> Monostable/1
  Constant2/1 -> Switch1/3
  Current/1 -> Main Relay/1("Three phase actual currents ")
  Counter1/2 -> Display2/1, Not3/1
  Main Relay/1(AR signal) -> Data  Conversion/1
  Monostable/1 -> Not5/1
  Delay/1 -> Sum/2
  Switch/1 -> Not4/1, Display4/1

== system Project/PROTECTION 3/overcurrent relay3 ==
  Current : Inport
  Constant : Constant
  Constant2 : Constant  Value=0
  Counter1 : dspswit3/Counter  Direction=Up  CountEvent=Rising edge  CounterSize=8 bits  MaxCount=255  InitialCount=0  Output=Count and Hit  HitValue=1  ResetInput=off  SamplesPerFrame=1  Ts=1  CntDtype=double  HitDtype=Logical
  Data  Conversion : DataTypeConversion  OutDataTypeStr=double
  Delay : Delay  DelayLength=1
  Display{2..6} (5 alike) : Display
  Main Relay : Subsystem
  Monostable : powerlib_meascontrol/Logic/Monostable  EdgeDetect=Rising  PulseDuration=.05  ic=0  Ts=0
      settings: SourceProductName=Simscape Power Systems  SourceProductBaseCode=PS
  Not{1,3..5} (4 alike) : Logic  Operator=NOT  IconShape=distinctive  AllPortsSameDT=off  OutDataTypeStr=boolean
  Scope2 : Scope
  Scope3 : Scope
  Sum : Sum  Inputs=|++
  Switch : Switch  Criteria=u2 > Threshold  Threshold=1
  Switch1 : Switch  Criteria=u2 > Threshold
  "CB control signal " : Outport
  wires:
  Constant/1 -> Main Relay/2("CT ratio ")
  Switch1/1 -> Not1/1, Scope2/1, "CB control signal "/1
  Sum/1 -> Counter1/1
  Not5/1 -> Switch1/1
  Not1/1 -> Delay/1
  Data  Conversion/1 -> Scope3/1, Display6/1, Switch/3, Display5/1, Sum/1
  Counter1/1 -> Display3/1, Switch/2
  Not3/1 -> Switch/1, Switch1/2
  Not4/1 -> Monostable/1
  Constant2/1 -> Switch1/3
  Current/1 -> Main Relay/1("Three phase actual currents ")
  Counter1/2 -> Display2/1, Not3/1
  Main Relay/1(AR signal) -> Data  Conversion/1
  Monostable/1 -> Not5/1
  Delay/1 -> Sum/2
  Switch/1 -> Not4/1, Display4/1

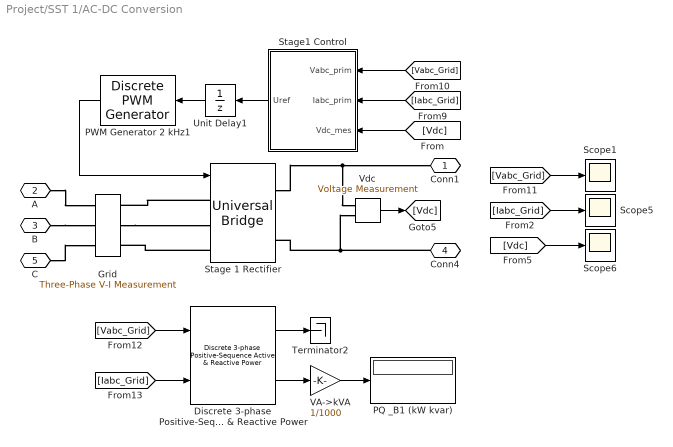
== system Project/SST 1/AC-DC Conversion ==
  Discrete 3-phase Positive-Sequence Active & Reactive Power : powerlib_extras/Discrete Measurements/Discrete 3-phase  Positive-Sequence  Active & Reactive Power  Freq=60  Par_Vinit=[0 0]  Par_Iinit=[0 0]  Ts=Ts
  Grid : powerlib/Measurements/Three-Phase V-I Measurement  VoltageMeasurement=phase-to-phase  SetLabelV=on  LabelV=Vabc_Grid  Vpu=off  VpuLL=off  CurrentMeasurement=yes  SetLabelI=on  LabelI=Iabc_Grid  Ipu=off  Pbase=100e6  Vbase=500e3  OutputType=Magnitude  PhasorSimulation=off  PSBequivalent=0
  PQ _B1 (kW kvar) : Display
      settings: Decimation=2000
  PWM Generator 2 kHz1 : powerlib_extras/Discrete  Control Blocks/Discrete PWM Generator  GeneratorMode="3-arm  bridge (6 pulses)"  Fc=2000  Ts=Ts  Internal=off  mIndex=0.4  Freq=60  Phase=0
  Scope1 : Scope
  Scope5 : Scope
  Scope6 : Scope
  Stage 1 Rectifier : powerlib/Power Electronics/Universal Bridge  Arms=3  SnubberResistance=1e5  SnubberCapacitance=inf  Device=IGBT / Diodes  Ron=1e-3  Lon=0  ForwardVoltages="[  0  0  ]"  ForwardVoltage=0  GTOparameters=[ 10e-6 , 20e-6 ]  IGBTparameters="[ 0  0  ]"  Measurements=None  Measurements_2=None  converterType=Rectifier
  Stage1 Control : Subsystem  mask(VSC Main Controller){nom=[ 50e3  60 ], Vnom=[ 4e3 1000 ], Vnom_dc=680, RLxfo=[0.008  0.04 ], RLchoke=[2e-3*(2*pi*60)/50   2e-3], K_VDCreg=[7  800], K_Ireg=[0.3 20]*1.5, Ts=Ts_Control}
      mask prompts: nom "Nominal power and frequency [ Pnom(VA)  Fnom(Hz) ]:"; Vnom "Nominal primary and secondary voltages (Vrms LL) [ Vnom_prim   Vnom_sec ]:"; Vnom_dc "Nominal DC bus voltage (V):"; RLxfo "Total transformer leakage impedance (pu/Pnom) [ Rxfo  Lxf ]"; RLchoke "Choke impedance [ R(ohm) L(H) ]"; K_VDCreg "VDC regultator gains [ Kp  Ki ]:"; K_Ireg "Current regulator gains [ Kp  Ki ]:"; Ts "Sample time"
      mask init:
      | Pnom=nom(1);
      | Fnom=nom(2);
      | Vnom_prim=Vnom(1);
      | Vnom_sec=Vnom(2);
      | Zbase=Vnom_sec^2/Pnom;
      | Rtot_pu=RLxfo(1) + RLchoke(1)/Zbase;
      | Ltot_pu=RLxfo(2) + RLchoke(2)/(Zbase/(2*pi*Fnom));
      | Kp_VDCreg=K_VDCreg(1);
      | Ki_VDCreg=K_VDCreg(2);
      | Kp_Ireg=K_Ireg(1);
      | Ki_Ireg=K_Ireg(2);
      | Vdc_ref=Vnom_dc;
      | % Used to determine initial value of Boost Control (MPPT)
      | assignin('base','Vdc_ref_Inv',Vdc_ref);
  Terminator2 : Terminator
  Unit Delay1 : UnitDelay  SampleTime=Ts_Control
  VA->kVA : Gain  Gain=1/1000
  "Vdc " : powerlib/Measurements/Voltage Measurement  Tag=PoWeRsYsTeMmEaSuReMeNt  PhasorSimulation=off  OutputType=Magnitude  PSBequivalent=0
  Conn1 : PMIOPort  Side=Right
  A : PMIOPort  Port=2  Side=Left
  B : PMIOPort  Port=3  Side=Left
  Conn4 : PMIOPort  Port=4  Side=Right
  C : PMIOPort  Port=5  Side=Left
  wires:
  [Vdc] -> Scope6/1
  [Vabc_Grid] -> Discrete 3-phase Positive-Sequence Active & Reactive Power/1
  [Iabc_Grid] -> Scope5/1
  [Iabc_Grid] -> Stage1 Control/2(Iabc_prim)
  "Vdc "/1 -> [Vdc]
  [Iabc_Grid] -> Discrete 3-phase Positive-Sequence Active & Reactive Power/2
  Stage1 Control/1(Uref) -> Unit Delay1/1
  Discrete 3-phase Positive-Sequence Active & Reactive Power/2 -> VA->kVA/1
  PWM Generator 2 kHz1/1 -> Stage 1 Rectifier/1
  VA->kVA/1 -> PQ _B1 (kW kvar)/1
  Discrete 3-phase Positive-Sequence Active & Reactive Power/1 -> Terminator2/1
  [Vdc] -> Stage1 Control/3(Vdc_mes)
  [Vabc_Grid] -> Stage1 Control/1(Vabc_prim)
  Unit Delay1/1 -> PWM Generator 2 kHz1/1
  [Vabc_Grid] -> Scope1/1
  connections:
  Stage 1 Rectifier/RConn2 -- "Vdc "/LConn2 -- Conn4/RConn1
  Stage 1 Rectifier/LConn1 -- Grid/RConn1
  Grid/RConn2 -- Stage 1 Rectifier/LConn2
  Stage 1 Rectifier/RConn1 -- "Vdc "/LConn1 -- Conn1/RConn1
  Stage 1 Rectifier/LConn3 -- Grid/RConn3
  C/RConn1 -- Grid/LConn3
  A/RConn1 -- Grid/LConn1
  B/RConn1 -- Grid/LConn2
